simulink model "heli_q8"  (R2014a)
settings: Solver=ode1  StartTime=0.0  StopTime=inf  FixedStep=0.002  RelTol=1e-3
PostLoadFcn:
  | qc_set_target_type(getConfigSet(bdroot, 'QUARC Default Target Configuration'));
values from neighbouring files (symbols this model uses):
  A_p4p2 = [0 0 0 0 0 -0.926877316308 1 0 0 0 0 0 ... (36 elements, 6x6)]    [heli_v5.mat]    (also in init_heli.m = [)
  B_p4p2 = [0  0; 0  0.61746031746; 0  0; 0.0993637376927  0; 0  0; 0  0]    [heli_v5.mat]    (also in init_heli.m = [)
  C_p4p2 = [1 0 0 0 0 0 0 1 0 0 0 0 ... (18 elements, 3x6)]    [heli_v5.mat]    (also in init_heli.m = [)
  Joystick_gain_x = 1    [heli.mat]    (also in heli_v2.mat; heli_v3.mat; heli_v4.mat; heli_v5.mat)
  Joystick_gain_y = -1    [heli.mat]    (also in heli_v2.mat; heli_v3.mat; heli_v4.mat; heli_v5.mat)
  K_p3p2 = [0  0  10; 3.16227766017  3.35303639847  0]    [heli_v4.mat]    (also in heli_v5.mat = [0  0  31.6227766017; 3.16227766017  3.35303639847  0]; init_heli.m = lqr(A_p3p1,B_p3p1,Q_p3p2,R_p3p2))
  K_p3p3 = [3.11100011502e-16  -3.0775394805e-16  10.9602950373  -3.30376513683e-16  -1; 4.20040589293  3.82170483266  -1.91242655394e-15  -1  -1.23212746659e-16]    [heli_v4.mat]    (also in heli_v5.mat = [-5.30623224306e-17  4.08389146172e-16  32.3265792615  1.739; init_heli.m = lqr(A_p3p3,B_p3p3,Q_p3p3,R_p3p3))
  K_pd = 1    [heli_v2.mat]    (also in heli_v3.mat = 11.6606683805; heli_v4.mat = 11.6606683805; heli_v5.mat = 11.6606683805; matlab_v4.mat = 11.6606683805)
  K_pp = 1    [heli_v2.mat]    (also in heli_v3.mat = 20.9892030848; heli_v4.mat = 20.9892030848; heli_v5.mat = 20.9892030848; matlab_v4.mat = 20.9892030848)
  K_rp = 10    [heli_v3.mat]    (also in heli_v4.mat = 3; heli_v5.mat = 3; matlab_v4.mat = 3)
  L = [5.92554151514 9.30695114405 0.0303026409954 -0.158988846376 1.02705256088 2.3799077818 0.00310751540277 -0.175228041509 6.12526482605 9.80708337963 0.209399631745 0.659991765117 ... (18 elements, 6x3)]    [heli_v5.mat]    (also in init_heli.m = place(A_p4p2',C_p4p2',poles).')
  P_p3p2 = [0  10; 3.16227766017  0]    [heli_v4.mat]    (also in heli_v5.mat = [0  31.6227766017; 3.16227766017  0]; init_heli.m = inv(C_p3p1*inv(B_p3p1*K_p3p2-A_p3p1)*B_p3p1))
  P_p3p3 = [9.92153997111  9.06487564165e+16; 2.9174989874e+16  35.9409347137]    [heli_v4.mat]    (also in heli_v5.mat = [-5.30623224306e-17  32.3265792615; 3.49573681243  2.5377879; init_heli.m = inv(C_p3p1*inv(B_p3p1*K_p3p3(1:2,1:3) - A_p3p1)*B_p3p1))
  V_zero_offset = 6.4201    [heli_v4.mat]    (also in heli_v5.mat; init_heli.m)
undefined symbols (not defined in the file or in its folder): HIL, qc_get_step_size
libraries: simulink x9, simulink_extras x6, quarc_library x4
settings Model: SimulationMode=external  ExtModeTrigDuration=5000  Creator=Rchan  LastModifiedBy=magho
settings SolverCC: PositivePriorityOrder=on
settings DataIOCC: SignalLoggingSaveFormat=ModelDataLogs
settings OptimizationCC: ExpressionDepthLimit=2147483647  InitFltsAndDblsToZero=on
settings DebuggingCC: SaveWithParameterizedLinksMsg=none  UnderspecifiedInitializationDetection=Classic  MultiTaskDSMMsg=warning  MultiTaskCondExecSysMsg=none  MultiTaskRateTransMsg=warning  FcnCallInpInsideContextMsg=UseLocalSettings  StateNameClashWarn=warning
settings RTWCC: SystemTargetFile=quarc_win64.tlc  TemplateMakefile=quarc_default_tmf  Description=QUARC Win64 Target  ProcessScript=quarc_win64_make_rtw_hook
settings STFCustomTargetCC: CPPClassGenCompliant=on
settings GRTTargetCC: ParMdlRefBuildCompliant=off  CompOptLevelCompliant=off  CombineOutputUpdateFcns=off  MatFileLogging=off  GRTInterface=on  ExtMode=on  ExtModeMexFile=quarc_comm

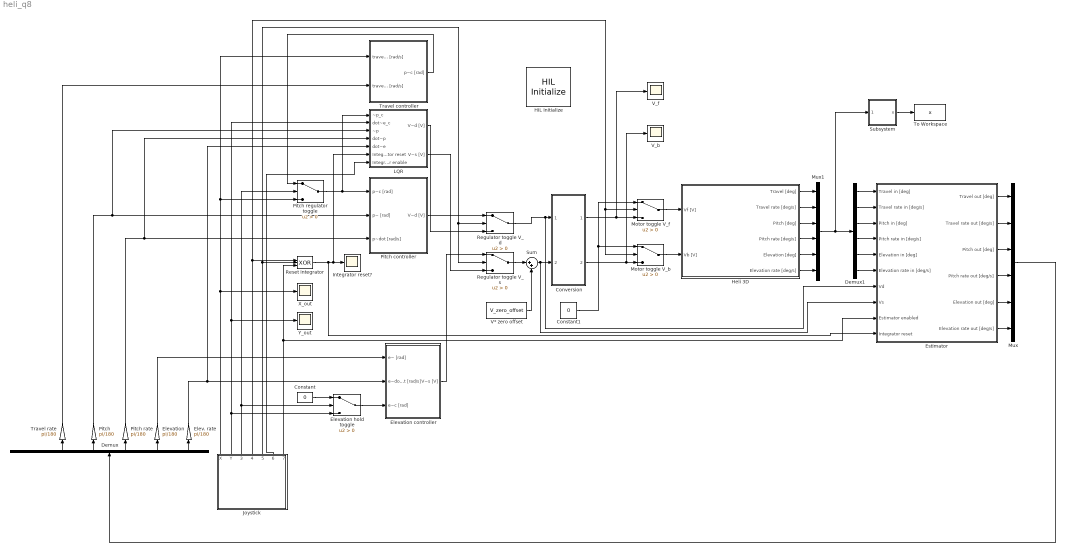
== system heli_q8 ==
  Constant : Constant  Value=0
  Constant1 : Constant  Value=0
  Conversion : Subsystem
  Demux : Demux  Outputs=6
  Demux1 : Demux  Outputs=6
  Elev. rate : Gain  Gain=pi/180
  Elevation : Gain  Gain=pi/180
  Elevation controller : Subsystem
  Elevation hold toggle : Switch  Criteria=u2 > Threshold
  Estimator : Subsystem
  HIL Initialize : quarc_library/Data Acquisition/Generic/Configuration/HIL Initialize  Priority=-99  object_name=HIL-1  board_type=q8_usb  board_number=0  board_options=update_rate=normal;decimation=1  exclusive=off  active=off  hardware_clocks=[0:2]  clock_modes=[]  initial_clock_frequencies=[]  set_clock_params_at_start=off  set_clock_params_at_switch_in=off  set_clock_frequencies_at_start=off  set_clock_frequencies_at_switch_in=off  analog_input_channels=[0:7]  analog_input_maximums=10  analog_input_minimums=-10  set_analog_input_params_at_start=on  set_analog_input_params_at_switch_in=off  analog_output_channels=[0:7]  analog_output_maximums=10  analog_output_minimums=-10  initial_analog_outputs=[0]  final_analog_outputs=[0]  watchdog_analog_outputs=0  set_analog_output_params_at_start=on  set_analog_output_params_at_switch_in=off  set_analog_outputs_at_start=on  set_analog_outputs_at_switch_in=off  set_analog_outputs_at_terminate=on  set_analog_outputs_at_switch_out=off  set_analog_outputs_on_watchdog=off  digital_input_channels=[]  digital_output_channels=[]  digital_output_configuration=[]  initial_digital_outputs=[1]  final_digital_outputs=[1]  watchdog_digital_outputs=[1]  set_digital_output_params_at_start=off  set_digital_output_params_at_switch_in=off  set_digital_outputs_at_start=on  set_digital_outputs_at_switch_in=off  set_digital_outputs_at_terminate=on  set_digital_outputs_at_switch_out=off  set_digital_outputs_on_watchdog=off  encoder_channels=[0:7]  quadrature=[4]  encoder_filter_frequency=[]  initial_encoder_counts=[0]  set_encoder_params_at_start=on  set_encoder_params_at_switch_in=off  set_encoder_counts_at_start=on  set_encoder_counts_at_switch_in=off  pwm_channels=[0:7]  pwm_modes=0  pwm_frequency=99.532799999999995e6/4095  pwm_configuration=[0]  pwm_alignment=[0]  pwm_polarity=[1]  pwm_leading_deadband=[0]  pwm_trailing_deadband=[0]  initial_pwm_outputs=[0]  final_pwm_outputs=[0]  watchdog_pwm_outputs=[0]  set_pwm_params_at_start=on  set_pwm_params_at_switch_in=off  set_pwm_outputs_at_start=on  set_pwm_outputs_at_switch_in=off  set_pwm_outputs_at_terminate=on  set_pwm_outputs_at_switch_out=off  set_pwm_outputs_on_watchdog=off  other_output_channels=[]  initial_other_outputs=[]  final_other_outputs=[]  watchdog_other_outputs=[]  set_other_outputs_at_start=off  set_other_outputs_at_switch_in=off  set_other_outputs_at_terminate=off  set_other_outputs_at_switch_out=off  set_other_outputs_on_watchdog=off
  Heli 3D : Subsystem
  Integrator reset? : Scope
      settings: TimeRange=10  YMin=-1  YMax=6.5  SaveName=ScopeData18
  Joystick : Subsystem
  LQR : Subsystem
  Motor toggle V_b : Switch  Criteria=u2 > Threshold
  Motor toggle V_f : Switch  Criteria=u2 > Threshold
  Mux : Mux  Inputs=6
  Mux1 : Mux  Inputs=6
  Pitch : Gain  Gain=pi/180
  Pitch controller : Subsystem
  Pitch rate : Gain  Gain=pi/180
  Pitch regulator toggle : Switch  Criteria=u2 > Threshold
  Regulator toggle V_d : Switch  Criteria=u2 > Threshold
  Regulator toggle V_s : Switch  Criteria=u2 > Threshold
  Reset integrator : Logic  Operator=XOR  Inputs=3  AllPortsSameDT=off  OutDataTypeStr=boolean
  Subsystem : Subsystem
  Sum : Sum  Inputs=|++
  To Workspace : ToWorkspace  VariableName=x  SaveFormat=Structure With Time  SampleTime=-1
  Travel controller : Subsystem
  Travel rate : Gain  Gain=pi/180
  "V* zero offset " : Constant  Value=V_zero_offset
  V_b : Scope
      settings: YMin=-7e+16  YMax=8e+16  SaveName=ScopeData17
  V_f : Scope
      settings: YMin=0  YMax=1.8e+15  SaveName=ScopeData16
  X_out : Scope
      settings: TimeRange=10  YMin=-1  YMax=6.5
  Y_out : Scope
      settings: YMax=8
  wires:
  Joystick/2(Y) -> Elevation hold toggle/3, Y_out/1, LQR/2(dot~e_c)
  Elev. rate/1 -> LQR/5(dot~e), Elevation controller/2(e~dot [rad/s])
  Elevation/1 -> Elevation controller/1(e~ [rad])
  Elevation controller/1(V~s [V]) -> Regulator toggle V_s/1
  Pitch/1 -> LQR/3(~p), Pitch controller/2(p~ [rad])
  Pitch rate/1 -> LQR/4(dot~p), Pitch controller/3(p~dot [rad/s])
  Constant/1 -> Elevation hold toggle/1
  Elevation hold toggle/1 -> Elevation controller/3(e~c [rad])
  Joystick/3(Travel Regulator Toggle) -> Elevation hold toggle/2, Pitch regulator toggle/2
  Pitch regulator toggle/1 -> Pitch controller/1(p~c [rad]), LQR/1(~p_c)
  Joystick/1(X) -> X_out/1, Pitch regulator toggle/3, Travel controller/1(travel rate_c [rad/s])
  Travel rate/1 -> Travel controller/2(travel rate [rad/s])
  Travel controller/1(p~c [rad]) -> Pitch regulator toggle/1
  Motor toggle V_b/1 -> Heli 3D/2(Vb [V])
  Motor toggle V_f/1 -> Heli 3D/1(Vf [V])
  Joystick/4(Motor Toggle) -> Motor toggle V_b/2, Motor toggle V_f/2, Reset integrator/1
  Conversion/2(Vb [V]) -> V_b/1, Motor toggle V_b/3
  Conversion/1(Vf [V]) -> V_f/1, Motor toggle V_f/3
  Constant1/1 -> Motor toggle V_f/1, Motor toggle V_b/1
  Regulator toggle V_d/1 -> Estimator/7(Vd), Conversion/1(Vd [V])
  Pitch controller/1(V~d [V]) -> Regulator toggle V_d/1
  Joystick/5(LQR toggle) -> Regulator toggle V_s/2, Regulator toggle V_d/2, Reset integrator/2
  LQR/2(V~s [V]) -> Regulator toggle V_s/3
  LQR/1(V~d [V]) -> Regulator toggle V_d/3
  Sum/1 -> Estimator/8(Vs), Conversion/2(Vs [V])
  Regulator toggle V_s/1 -> Sum/1
  "V* zero offset "/1 -> Sum/2
  Mux/1 -> Demux/1
  Demux/3 -> Pitch/1
  Demux/4 -> Pitch rate/1
  Demux/5 -> Elevation/1
  Demux/2 -> Travel rate/1
  Demux/6 -> Elev. rate/1
  Reset integrator/1 -> LQR/6(Integrator reset), Integrator reset?/1, Estimator/10(Integrator reset)
  Joystick/6(LQR integrator toggle) -> LQR/7(Integrator enable)
  Estimator/1(Travel out [deg]) -> Mux/1
  Estimator/3(Pitch out [deg]) -> Mux/3
  Estimator/4(Pitch rate out [deg/s]) -> Mux/4
  Estimator/5(Elevation out [deg]) -> Mux/5
  Estimator/6(Elevation rate out [deg/s]) -> Mux/6
  Estimator/2(Travel rate out [deg/s]) -> Mux/2
  Joystick/7(Estimator toggle) -> Reset integrator/3, Estimator/9("Estimator enabled ")
  Heli 3D/1(Travel [deg]) -> Mux1/1
  Heli 3D/2(Travel rate [deg/s]) -> Mux1/2
  Heli 3D/3(Pitch [deg]) -> Mux1/3
  Heli 3D/4(Pitch rate [deg/s]) -> Mux1/4
  Heli 3D/5(Elevation [deg]) -> Mux1/5
  Heli 3D/6(Elevation rate [deg/s]) -> Mux1/6
  Demux1/1 -> Estimator/1(Travel in [deg])
  Demux1/2 -> Estimator/2(Travel rate in [deg/s])
  Demux1/3 -> Estimator/3(Pitch in [deg])
  Demux1/4 -> Estimator/4(Pitch rate in [deg/s])
  Demux1/5 -> Estimator/5(Elevation in [deg])
  Demux1/6 -> Estimator/6(Elevation rate in [deg/s])
  Mux1/1 -> Subsystem/1(x_weird), Demux1/1
  Subsystem/1(x) -> To Workspace/1

== system heli_q8/Conversion ==
  Vd [V] : Inport
  Vs [V] : Inport  Port=2
  Add : Sum
  Back gain : Gain  Gain=0.5
  Front gain : Gain  Gain=0.5
  Subtract : Sum  Inputs=+-
  Vf [V] : Outport
  Vb [V] : Outport  Port=2
  wires:
  Vd [V]/1 -> Subtract/2, Add/1
  Vs [V]/1 -> Subtract/1, Add/2
  Subtract/1 -> Back gain/1
  Back gain/1 -> Vb [V]/1
  Add/1 -> Front gain/1
  Front gain/1 -> Vf [V]/1

== system heli_q8/Elevation controller ==
  e~ [rad] : Inport
  e~dot [rad/s] : Inport  Port=2
  e~c [rad] : Inport  Port=3
  Elevation controller : Subsystem
  Sum : Sum  Inputs=-+  SaturateOnIntegerOverflow=on  InputSameDT=on  OutDataTypeStr=Inherit: Same as first input
  V~s [V] : Outport  InitialOutput=0
  wires:
  Sum/1 -> Elevation controller/1(e~ [rad])
  Elevation controller/1(V~_s [V]) -> V~s [V]/1
  e~ [rad]/1 -> Sum/1
  e~dot [rad/s]/1 -> Elevation controller/2(e~_dot [rad/s])
  e~c [rad]/1 -> Sum/2

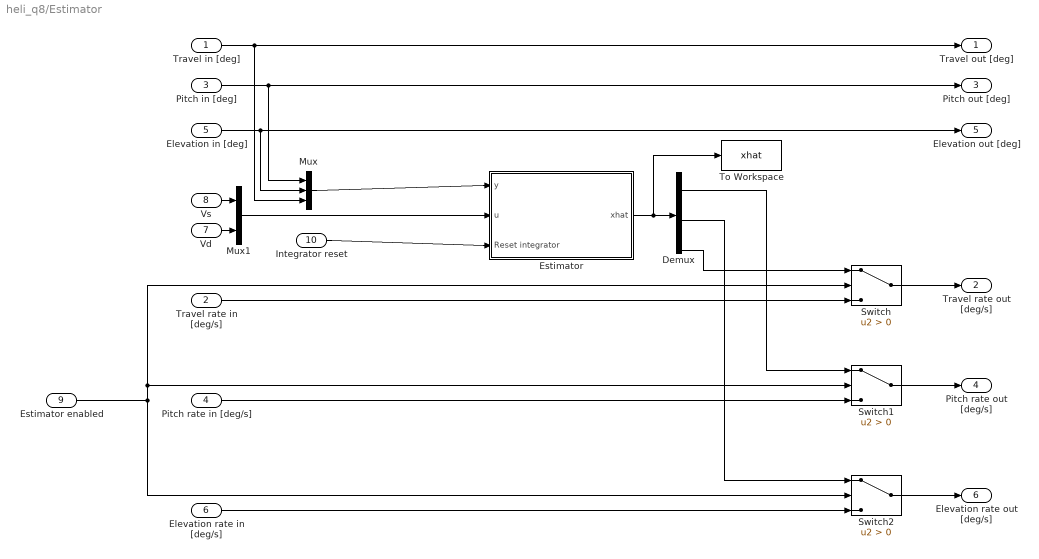
== system heli_q8/Estimator ==
  Travel in [deg] : Inport
  Travel rate in [deg/s] : Inport  Port=2
  Pitch in [deg] : Inport  Port=3
  Pitch rate in [deg/s] : Inport  Port=4
  Elevation in [deg] : Inport  Port=5
  Elevation rate in [deg/s] : Inport  Port=6
  Vd : Inport  Port=7
  Vs : Inport  Port=8
  "Estimator enabled " : Inport  Port=9
  Integrator reset : Inport  Port=10
  Demux : Demux  Outputs=6
  Estimator : Subsystem
  Mux : Mux  Inputs=3
  Mux1 : Mux  Inputs=2
  Switch : Switch  Criteria=u2 > Threshold
  Switch1 : Switch  Criteria=u2 > Threshold
  Switch2 : Switch  Criteria=u2 > Threshold
  To Workspace : ToWorkspace  VariableName=xhat  SaveFormat=Structure With Time  SampleTime=-1
  Travel out [deg] : Outport
  Travel rate out [deg/s] : Outport  Port=2
  Pitch out [deg] : Outport  Port=3
  Pitch rate out [deg/s] : Outport  Port=4
  Elevation out [deg] : Outport  Port=5
  Elevation rate out [deg/s] : Outport  Port=6
  wires:
  Travel in [deg]/1 -> Travel out [deg]/1, Mux/3
  Pitch in [deg]/1 -> Mux/1, Pitch out [deg]/1
  Elevation in [deg]/1 -> Elevation out [deg]/1, Mux/2
  Travel rate in [deg/s]/1 -> Switch/3
  Pitch rate in [deg/s]/1 -> Switch1/3
  Elevation rate in [deg/s]/1 -> Switch2/3
  Switch1/1 -> Pitch rate out [deg/s]/1
  Switch/1 -> Travel rate out [deg/s]/1
  Switch2/1 -> Elevation rate out [deg/s]/1
  "Estimator enabled "/1 -> Switch2/2, Switch/2, Switch1/2
  Mux/1 -> Estimator/1(y)
  Integrator reset/1 -> Estimator/3(Reset integrator)
  Vd/1 -> Mux1/2
  Vs/1 -> Mux1/1
  Mux1/1 -> Estimator/2(u)
  Estimator/1(xhat) -> To Workspace/1, Demux/1
  Demux/2 -> Switch1/1
  Demux/4 -> Switch2/1
  Demux/6 -> Switch/1

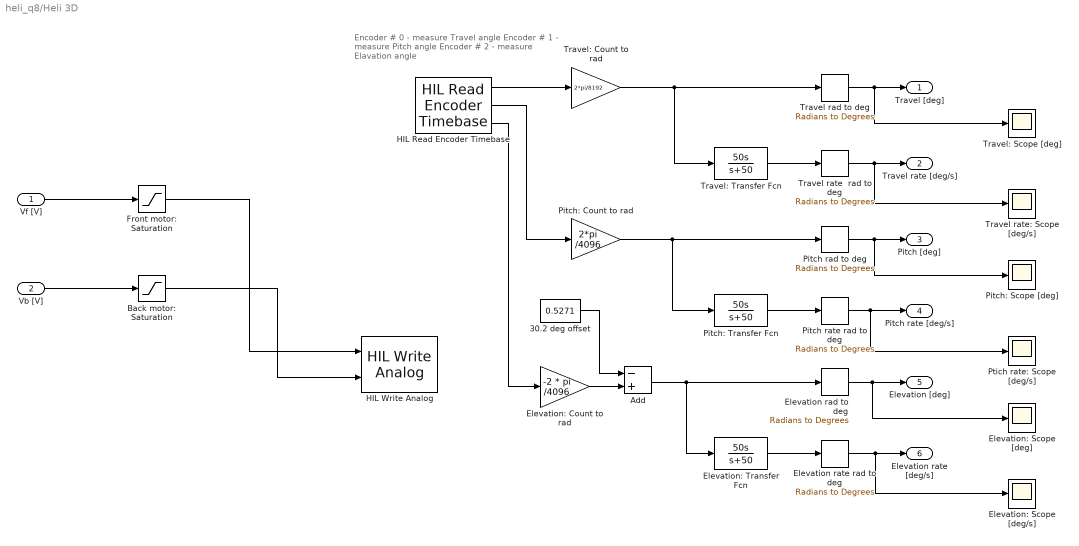
== system heli_q8/Heli 3D ==
  note: Encoder # 0 - measure Travel angle
      | Encoder # 1 - measure Pitch angle
      | Encoder # 2 - measure Elavation angle
  Vf [V] : Inport
  Vb [V] : Inport  Port=2
  30.2 deg offset : Constant  Value=0.5271
  Add : Sum  Inputs=-+
  Back motor: Saturation : Saturate  UpperLimit=5  LowerLimit=-5
  Elevation rad to deg : simulink_extras/Transformations/Radians to Degrees
  Elevation rate rad to deg : simulink_extras/Transformations/Radians to Degrees
  Elevation: Count to rad : Gain  Gain=-2 * pi /4096
  Elevation: Scope [deg/s] : Scope
      settings: YMin=-15  YMax=15  SaveName=ScopeData13
  Elevation: Scope [deg] : Scope
      settings: YMin=-32.5  YMax=0  SaveName=ScopeData12
  Elevation: Transfer Fcn : TransferFcn  Numerator=[50 0]  Denominator=[1 50]
  Front motor: Saturation : Saturate  UpperLimit=5  LowerLimit=-5
  HIL Read Encoder Timebase : quarc_library/Data Acquisition/Generic/Timebases/HIL Read Encoder Timebase  object_name=HIL-1  clock=0  channels=[0:2]  samples_in_buffer=max(ceil(1/qc_get_step_size), 1)  active=on  vector_output=off  data_type_mode=Inherit via back propagation  data_type=double
  HIL Write Analog : quarc_library/Data Acquisition/Generic/Immediate I//O/HIL Write Analog  object_name=HIL-1  channels=[0:1]  sample_time=-1  active=off  vector_input=off
  Pitch rad to deg : simulink_extras/Transformations/Radians to Degrees
  Pitch rate rad to deg : simulink_extras/Transformations/Radians to Degrees
  Pitch: Count to rad : Gain  Gain=2*pi /4096
  Pitch: Scope [deg] : Scope
      settings: YMin=-0.3  YMax=1  SaveName=ScopeData10
  Pitch: Transfer Fcn : TransferFcn  Numerator=[50 0]  Denominator=[1 50]
  Ptich rate: Scope [deg/s] : Scope
      settings: YMin=-15  YMax=15  SaveName=ScopeData11
  Travel rad to deg : simulink_extras/Transformations/Radians to Degrees
  Travel rate  rad to deg : simulink_extras/Transformations/Radians to Degrees
  Travel rate: Scope [deg/s] : Scope
      settings: YMin=-3.5  YMax=3  SaveName=ScopeData9
  Travel: Count to rad : Gain  Gain=2*pi/8192
  Travel: Scope [deg] : Scope
      settings: YMin=-2.75  YMax=0.5  SaveName=ScopeData8
  Travel: Transfer Fcn : TransferFcn  Numerator=[50 0]  Denominator=[1 50]
  Travel [deg] : Outport
  Travel rate [deg/s] : Outport  Port=2
  Pitch [deg] : Outport  Port=3
  Pitch rate [deg/s] : Outport  Port=4
  Elevation [deg] : Outport  Port=5
  Elevation rate [deg/s] : Outport  Port=6
  wires:
  HIL Read Encoder Timebase/1 -> Travel: Count to rad/1
  HIL Read Encoder Timebase/2 -> Pitch: Count to rad/1
  Travel: Count to rad/1 -> Travel: Transfer Fcn/1, Travel rad to deg/1
  Travel: Transfer Fcn/1 -> Travel rate  rad to deg/1
  Pitch: Count to rad/1 -> Pitch: Transfer Fcn/1, Pitch rad to deg/1
  Pitch: Transfer Fcn/1 -> Pitch rate rad to deg/1
  Elevation: Transfer Fcn/1 -> Elevation rate rad to deg/1
  Travel rad to deg/1 -> Travel: Scope [deg]/1, Travel [deg]/1
  Travel rate  rad to deg/1 -> Travel rate: Scope [deg/s]/1, Travel rate [deg/s]/1
  Pitch rad to deg/1 -> Pitch: Scope [deg]/1, Pitch [deg]/1
  Pitch rate rad to deg/1 -> Ptich rate: Scope [deg/s]/1, Pitch rate [deg/s]/1
  Elevation rad to deg/1 -> Elevation: Scope [deg]/1, Elevation [deg]/1
  Elevation rate rad to deg/1 -> Elevation: Scope [deg/s]/1, Elevation rate [deg/s]/1
  Vf [V]/1 -> Front motor: Saturation/1
  Vb [V]/1 -> Back motor: Saturation/1
  Front motor: Saturation/1 -> HIL Write Analog/1
  Back motor: Saturation/1 -> HIL Write Analog/2
  HIL Read Encoder Timebase/3 -> Elevation: Count to rad/1
  Elevation: Count to rad/1 -> Add/2
  Add/1 -> Elevation rad to deg/1, Elevation: Transfer Fcn/1
  30.2 deg offset/1 -> Add/1

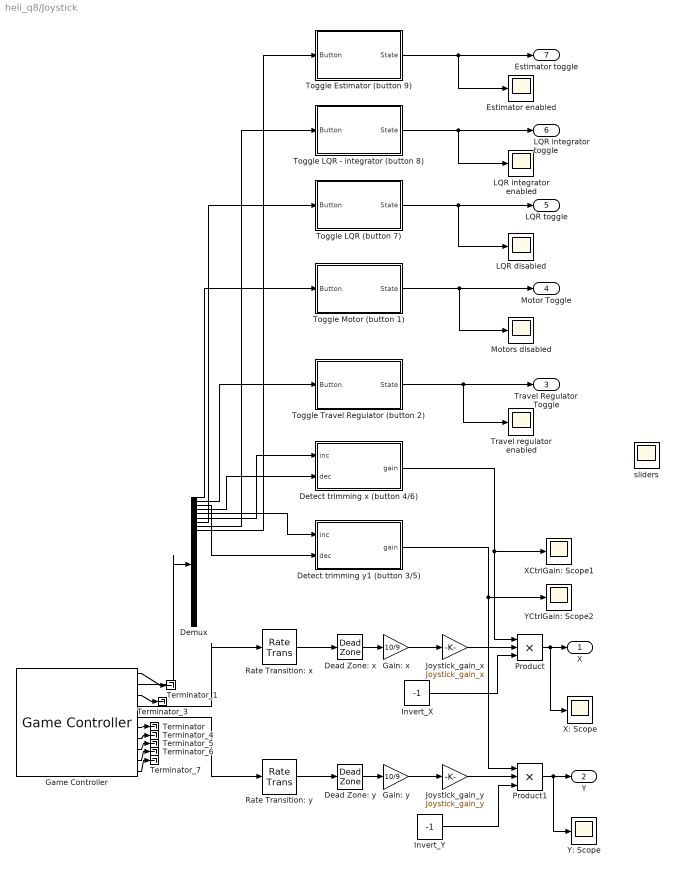
== system heli_q8/Joystick ==
  Dead Zone: x : DeadZone  LowerValue=-0.1  UpperValue=0.1  SaturateOnIntegerOverflow=on
  Dead Zone: y : DeadZone  LowerValue=-0.1  UpperValue=0.1  SaturateOnIntegerOverflow=on
  Demux : Demux  Outputs=32
  Detect trimming x (button 4/6) : Subsystem
  Detect trimming y1 (button 3/5) : Subsystem
  Estimator enabled : Scope
      settings: YMin=0.95  YMax=1.05  SaveName=ScopeData22
  Gain: x : Gain  Gain=10/9
  Gain: y : Gain  Gain=10/9
  Game Controller : quarc_library/Devices/Peripherals/Target/Game Controller  controller=1  buffer_size=12  deadzone=[]  saturation=[]  sample_time=max(qc_get_step_size, 0.01)  auto_center=off  enabled=on
  Invert_X : Constant  Value=-1
  Invert_Y : Constant  Value=-1
  Joystick_gain_x : Gain  Gain=Joystick_gain_x
  Joystick_gain_y : Gain  Gain=Joystick_gain_y
  LQR disabled : Scope
      settings: YMin=0.95  YMax=1.05  SaveName=ScopeData15
  LQR integrator enabled : Scope
      settings: YMin=0.95  YMax=1.05  SaveName=ScopeData21
  Motors disabled : Scope
      settings: YMin=0.95  YMax=1.05  SaveName=ScopeData6
  Product : Product  Inputs=3
  Product1 : Product  Inputs=3
  Rate Transition: x : RateTransition
  Rate Transition: y : RateTransition
  Terminator : Terminator
  Terminator_{1,3..7} (6 alike) : Terminator
  Toggle Estimator (button 9) : Subsystem
  Toggle LQR (button 7) : Subsystem
  Toggle LQR - integrator (button 8) : Subsystem
  Toggle Motor (button 1) : Subsystem
  Toggle Travel Regulator (button 2) : Subsystem
  Travel regulator enabled : Scope
      settings: YMin=0.95  YMax=1.05  SaveName=ScopeData14
  X: Scope : Scope
      settings: YMin=-1  YMax=1  SaveName=ScopeData7
  XCtrlGain: Scope1 : Scope
      settings: YMin=0  YMax=10  SaveName=ScopeData3
  Y: Scope : Scope
      settings: YMin=-10  YMax=10  SaveName=ScopeData5
  YCtrlGain: Scope2 : Scope
      settings: YMin=0  YMax=1.75  SaveName=ScopeData4
  sliders : Scope
      settings: YMin=-1  YMax=1  SaveName=ScopeData2
  X : Outport
  Y : Outport  Port=2
  Travel Regulator Toggle : Outport  Port=3
  Motor Toggle : Outport  Port=4
  LQR toggle : Outport  Port=5
  LQR integrator toggle : Outport  Port=6
  Estimator toggle : Outport  Port=7
  wires:
  Rate Transition: y/1 -> Dead Zone: y/1
  Rate Transition: x/1 -> Dead Zone: x/1
  Game Controller/5 -> Rate Transition: y/1
  Game Controller/4 -> Rate Transition: x/1
  Game Controller/1 -> Terminator_1/1
  Game Controller/7 -> Terminator_4/1
  Game Controller/8 -> Terminator_5/1
  Game Controller/9 -> Terminator_6/1
  Game Controller/10 -> Terminator_7/1
  Game Controller/6 -> Terminator/1
  Dead Zone: x/1 -> Gain: x/1
  Dead Zone: y/1 -> Gain: y/1
  Gain: x/1 -> Joystick_gain_x/1
  Gain: y/1 -> Joystick_gain_y/1
  Game Controller/2 -> Demux/1
  Game Controller/3 -> Terminator_3/1
  Joystick_gain_x/1 -> Product/2
  Detect trimming x (button 4/6)/1(gain) -> XCtrlGain: Scope1/1, Product/1
  Product/1 -> X: Scope/1, X/1
  Joystick_gain_y/1 -> Product1/2
  Product1/1 -> Y: Scope/1, Y/1
  Detect trimming y1 (button 3/5)/1(gain) -> Product1/1, YCtrlGain: Scope2/1
  Invert_X/1 -> Product/3
  Demux/6 -> Detect trimming x (button 4/6)/1(inc)
  Demux/4 -> Detect trimming x (button 4/6)/2(dec)
  Demux/5 -> Detect trimming y1 (button 3/5)/1(inc)
  Demux/3 -> Detect trimming y1 (button 3/5)/2(dec)
  Invert_Y/1 -> Product1/3
  Demux/1 -> Toggle Motor (button 1)/1(Button)
  Toggle Travel Regulator (button 2)/1(State) -> Travel regulator enabled/1, Travel Regulator Toggle/1
  Demux/2 -> Toggle Travel Regulator (button 2)/1(Button)
  Toggle Motor (button 1)/1(State) -> Motors disabled/1, Motor Toggle/1
  Demux/7 -> Toggle LQR (button 7)/1(Button)
  Toggle LQR (button 7)/1(State) -> LQR disabled/1, LQR toggle/1
  Demux/8 -> Toggle LQR - integrator (button 8)/1(Button)
  Toggle LQR - integrator (button 8)/1(State) -> LQR integrator enabled/1, LQR integrator toggle/1
  Demux/9 -> Toggle Estimator (button 9)/1(Button)
  Toggle Estimator (button 9)/1(State) -> Estimator enabled/1, Estimator toggle/1

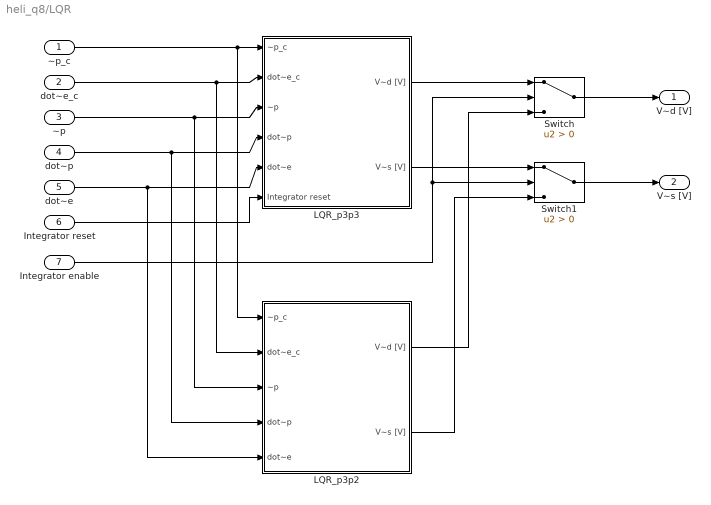
== system heli_q8/LQR ==
  ~p_c : Inport
  dot~e_c : Inport  Port=2
  ~p : Inport  Port=3
  dot~p : Inport  Port=4
  dot~e : Inport  Port=5
  Integrator reset : Inport  Port=6
  Integrator enable : Inport  Port=7
  LQR_p3p2 : Subsystem
  LQR_p3p3 : Subsystem
  Switch : Switch  Criteria=u2 > Threshold
  Switch1 : Switch  Criteria=u2 > Threshold
  V~d [V] : Outport
  V~s [V] : Outport  Port=2
  wires:
  ~p_c/1 -> LQR_p3p2/1(~p_c), LQR_p3p3/1(~p_c)
  dot~e_c/1 -> LQR_p3p2/2(dot~e_c), LQR_p3p3/2(dot~e_c)
  ~p/1 -> LQR_p3p2/3(~p), LQR_p3p3/3(~p)
  dot~p/1 -> LQR_p3p2/4(dot~p), LQR_p3p3/4(dot~p)
  dot~e/1 -> LQR_p3p2/5(dot~e), LQR_p3p3/5(dot~e)
  LQR_p3p3/1(V~d [V]) -> Switch/1
  Switch/1 -> V~d [V]/1
  Switch1/1 -> V~s [V]/1
  LQR_p3p3/2(V~s [V]) -> Switch1/1
  LQR_p3p2/1(V~d [V]) -> Switch/3
  LQR_p3p2/2(V~s [V]) -> Switch1/3
  Integrator reset/1 -> LQR_p3p3/6(Integrator reset)
  Integrator enable/1 -> Switch1/2, Switch/2

== system heli_q8/Pitch controller ==
  p~c [rad] : Inport
  p~ [rad] : Inport  Port=2
  p~dot [rad/s] : Inport  Port=3
  Add : Sum  Inputs=+-
  Add1 : Sum  Inputs=+-
  Gain : Gain  Gain=K_pp
  Gain1 : Gain  Gain=K_pd
  V~d [V] : Outport  InitialOutput=0
  wires:
  Add/1 -> V~d [V]/1
  p~dot [rad/s]/1 -> Gain1/1
  Gain1/1 -> Add/2
  p~c [rad]/1 -> Add1/1
  p~ [rad]/1 -> Add1/2
  Add1/1 -> Gain/1
  Gain/1 -> Add/1

== system heli_q8/Subsystem ==
  x_weird : Inport
  Demux2 : Demux  Outputs=6
  Mux2 : Mux  Inputs=6
  x : Outport
  wires:
  x_weird/1 -> Demux2/1
  Mux2/1 -> x/1
  Demux2/1 -> Mux2/5
  Demux2/2 -> Mux2/6
  Demux2/3 -> Mux2/1
  Demux2/4 -> Mux2/2
  Demux2/5 -> Mux2/3
  Demux2/6 -> Mux2/4

== system heli_q8/Travel controller ==
  travel rate_c [rad/s] : Inport
  travel rate [rad/s] : Inport  Port=2
  Add1 : Sum  Inputs=+-
  Gain : Gain  Gain=K_rp
  p~c [rad] : Outport  InitialOutput=0
  wires:
  Gain/1 -> p~c [rad]/1
  travel rate_c [rad/s]/1 -> Add1/2
  Add1/1 -> Gain/1
  travel rate [rad/s]/1 -> Add1/1

== system heli_q8/Elevation controller/Elevation controller ==
  e~ [rad] : Inport
  e~_dot [rad/s] : Inport  Port=2
  Integrator : Integrator  LimitOutput=on
  K_ed : Gain  Gain=12  SaturateOnIntegerOverflow=on  OutDataTypeStr=Inherit: Same as input  ParamDataTypeStr=Inherit: Same as input
  K_ei : Gain  Gain=5  SaturateOnIntegerOverflow=on  OutDataTypeStr=Inherit: Same as input  ParamDataTypeStr=Inherit: Same as input
  K_ep : Gain  Gain=15  SaturateOnIntegerOverflow=on  OutDataTypeStr=Inherit: Same as input  ParamDataTypeStr=Inherit: Same as input
  Sum : Sum  Inputs=++-  SaturateOnIntegerOverflow=on  InputSameDT=on  OutDataTypeStr=Inherit: Same as first input
  V~_s [V] : Outport  InitialOutput=0
  wires:
  K_ei/1 -> Integrator/1
  Integrator/1 -> Sum/1
  Sum/1 -> V~_s [V]/1
  e~_dot [rad/s]/1 -> K_ed/1
  K_ed/1 -> Sum/3
  K_ep/1 -> Sum/2
  e~ [rad]/1 -> K_ep/1, K_ei/1

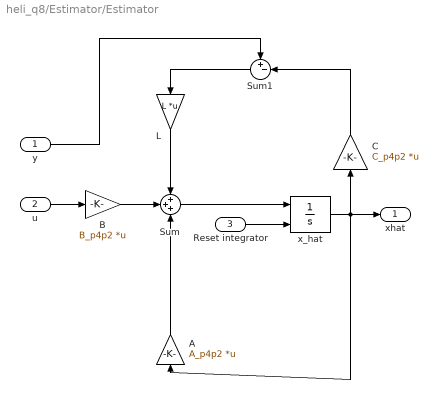
== system heli_q8/Estimator/Estimator ==
  y : Inport
  u : Inport  Port=2
  Reset integrator : Inport  Port=3
  A : Gain  Gain=A_p4p2  Multiplication=Matrix(K*u)
  B : Gain  Gain=B_p4p2  Multiplication=Matrix(K*u)
  C : Gain  Gain=C_p4p2  Multiplication=Matrix(K*u)
  L : Gain  Gain=L  Multiplication=Matrix(K*u)
  Sum : Sum  Inputs=+++
  Sum1 : Sum  Inputs=+-|
  x_hat : Integrator  ExternalReset=either
  xhat : Outport
  wires:
  x_hat/1 -> A/1, xhat/1, C/1
  Reset integrator/1 -> x_hat/2
  Sum/1 -> x_hat/1
  L/1 -> Sum/1
  y/1 -> Sum1/1
  C/1 -> Sum1/2
  Sum1/1 -> L/1
  A/1 -> Sum/3
  B/1 -> Sum/2
  u/1 -> B/1

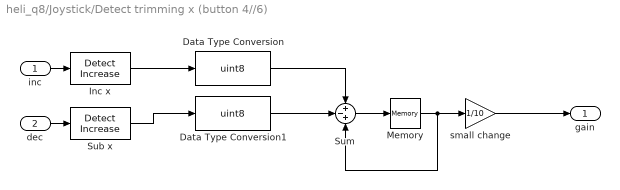
== system heli_q8/Joystick/Detect trimming x (button 4//6) ==
  inc : Inport
  dec : Inport  Port=2
  Data Type Conversion : DataTypeConversion  OutDataTypeStr=uint8
  Data Type Conversion1 : DataTypeConversion  OutDataTypeStr=uint8
  Inc x : simulink/Logic and Bit Operations/Detect Increase  vinit=0.0  InputProcessing=Inherited  OutDataTypeStr=boolean
  Memory : Memory  X0=20  InheritSampleTime=on
  Sub x : simulink/Logic and Bit Operations/Detect Increase  vinit=0.0  InputProcessing=Inherited  OutDataTypeStr=boolean
  Sum : Sum  Inputs=+-+
  small change : Gain  Gain=1/10
  gain : Outport
  wires:
  Sum/1 -> Memory/1
  Inc x/1 -> Data Type Conversion/1
  Memory/1 -> small change/1, Sum/3
  small change/1 -> gain/1
  Sub x/1 -> Data Type Conversion1/1
  inc/1 -> Inc x/1
  dec/1 -> Sub x/1
  Data Type Conversion/1 -> Sum/1
  Data Type Conversion1/1 -> Sum/2

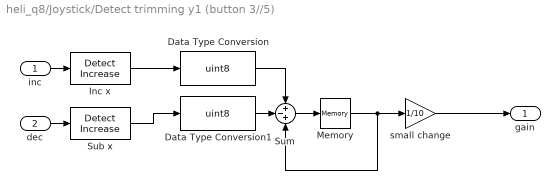
== system heli_q8/Joystick/Detect trimming y1 (button 3//5) ==
  inc : Inport
  dec : Inport  Port=2
  Data Type Conversion : DataTypeConversion  OutDataTypeStr=uint8
  Data Type Conversion1 : DataTypeConversion  OutDataTypeStr=uint8
  Inc x : simulink/Logic and Bit Operations/Detect Increase  vinit=0.0  InputProcessing=Inherited  OutDataTypeStr=boolean
  Memory : Memory  X0=15  InheritSampleTime=on
  Sub x : simulink/Logic and Bit Operations/Detect Increase  vinit=0.0  InputProcessing=Inherited  OutDataTypeStr=boolean
  Sum : Sum  Inputs=+-+
  small change : Gain  Gain=1/10
  gain : Outport
  wires:
  Sum/1 -> Memory/1
  Inc x/1 -> Data Type Conversion/1
  Memory/1 -> small change/1, Sum/3
  small change/1 -> gain/1
  Sub x/1 -> Data Type Conversion1/1
  inc/1 -> Inc x/1
  dec/1 -> Sub x/1
  Data Type Conversion/1 -> Sum/1
  Data Type Conversion1/1 -> Sum/2

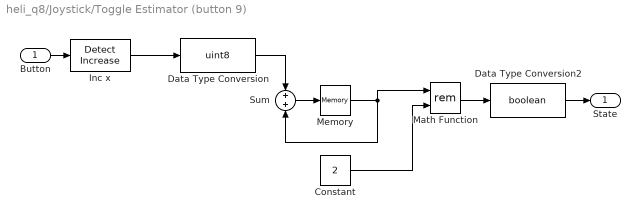
== system heli_q8/Joystick/Toggle Estimator (button 9) ==
  Button : Inport
  Constant : Constant  Value=2
  Data Type Conversion : DataTypeConversion  OutDataTypeStr=uint8
  Data Type Conversion2 : DataTypeConversion  OutDataTypeStr=boolean
  Inc x : simulink/Logic and Bit Operations/Detect Increase  vinit=0.0  InputProcessing=Inherited  OutDataTypeStr=boolean
  Math Function : Math  Operator=rem  SaturateOnIntegerOverflow=on
  Memory : Memory  X0=15  InheritSampleTime=on
  Sum : Sum
  State : Outport
  wires:
  Sum/1 -> Memory/1
  Inc x/1 -> Data Type Conversion/1
  Memory/1 -> Sum/2, Math Function/1
  Button/1 -> Inc x/1
  Data Type Conversion/1 -> Sum/1
  Constant/1 -> Math Function/2
  Math Function/1 -> Data Type Conversion2/1
  Data Type Conversion2/1 -> State/1

== system heli_q8/Joystick/Toggle LQR (button 7) ==
  Button : Inport
  Constant : Constant  Value=2
  Data Type Conversion : DataTypeConversion  OutDataTypeStr=uint8
  Data Type Conversion2 : DataTypeConversion  OutDataTypeStr=boolean
  Inc x : simulink/Logic and Bit Operations/Detect Increase  vinit=0.0  InputProcessing=Inherited  OutDataTypeStr=boolean
  Math Function : Math  Operator=rem  SaturateOnIntegerOverflow=on
  Memory : Memory  X0=15  InheritSampleTime=on
  Sum : Sum
  State : Outport
  wires:
  Sum/1 -> Memory/1
  Inc x/1 -> Data Type Conversion/1
  Memory/1 -> Sum/2, Math Function/1
  Button/1 -> Inc x/1
  Data Type Conversion/1 -> Sum/1
  Constant/1 -> Math Function/2
  Math Function/1 -> Data Type Conversion2/1
  Data Type Conversion2/1 -> State/1

== system heli_q8/Joystick/Toggle LQR - integrator (button 8) ==
  Button : Inport
  Constant : Constant  Value=2
  Data Type Conversion : DataTypeConversion  OutDataTypeStr=uint8
  Data Type Conversion2 : DataTypeConversion  OutDataTypeStr=boolean
  Inc x : simulink/Logic and Bit Operations/Detect Increase  vinit=0.0  InputProcessing=Inherited  OutDataTypeStr=boolean
  Math Function : Math  Operator=rem  SaturateOnIntegerOverflow=on
  Memory : Memory  X0=15  InheritSampleTime=on
  Sum : Sum
  State : Outport
  wires:
  Sum/1 -> Memory/1
  Inc x/1 -> Data Type Conversion/1
  Memory/1 -> Sum/2, Math Function/1
  Button/1 -> Inc x/1
  Data Type Conversion/1 -> Sum/1
  Constant/1 -> Math Function/2
  Math Function/1 -> Data Type Conversion2/1
  Data Type Conversion2/1 -> State/1

== system heli_q8/Joystick/Toggle Motor (button 1) ==
  Button : Inport
  Constant : Constant  Value=2
  Data Type Conversion : DataTypeConversion  OutDataTypeStr=uint8
  Data Type Conversion2 : DataTypeConversion  OutDataTypeStr=boolean
  Inc x : simulink/Logic and Bit Operations/Detect Increase  vinit=0.0  InputProcessing=Inherited  OutDataTypeStr=boolean
  Math Function : Math  Operator=rem  SaturateOnIntegerOverflow=on
  Memory : Memory  X0=15  InheritSampleTime=on
  Sum : Sum
  State : Outport
  wires:
  Sum/1 -> Memory/1
  Inc x/1 -> Data Type Conversion/1
  Memory/1 -> Sum/2, Math Function/1
  Button/1 -> Inc x/1
  Data Type Conversion/1 -> Sum/1
  Constant/1 -> Math Function/2
  Math Function/1 -> Data Type Conversion2/1
  Data Type Conversion2/1 -> State/1

== system heli_q8/Joystick/Toggle Travel Regulator (button 2) ==
  Button : Inport
  Constant : Constant  Value=2
  Data Type Conversion : DataTypeConversion  OutDataTypeStr=uint8
  Data Type Conversion2 : DataTypeConversion  OutDataTypeStr=boolean
  Inc x : simulink/Logic and Bit Operations/Detect Increase  vinit=0.0  InputProcessing=Inherited  OutDataTypeStr=boolean
  Math Function : Math  Operator=rem  SaturateOnIntegerOverflow=on
  Memory : Memory  X0=16  InheritSampleTime=on
  Sum : Sum
  State : Outport
  wires:
  Sum/1 -> Memory/1
  Inc x/1 -> Data Type Conversion/1
  Memory/1 -> Sum/2, Math Function/1
  Button/1 -> Inc x/1
  Data Type Conversion/1 -> Sum/1
  Constant/1 -> Math Function/2
  Math Function/1 -> Data Type Conversion2/1
  Data Type Conversion2/1 -> State/1

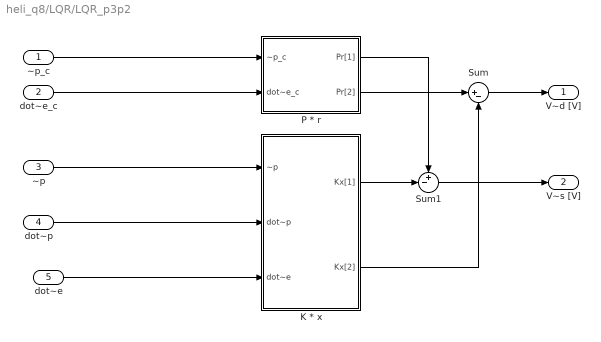
== system heli_q8/LQR/LQR_p3p2 ==
  ~p_c : Inport
  dot~e_c : Inport  Port=2
  ~p : Inport  Port=3
  dot~p : Inport  Port=4
  dot~e : Inport  Port=5
  K * x : Subsystem
  P * r : Subsystem
  Sum : Sum  Inputs=|+-
  Sum1 : Sum  Inputs=+-|
  V~d [V] : Outport
  V~s [V] : Outport  Port=2
  wires:
  dot~p/1 -> K * x/2(dot~p)
  ~p/1 -> K * x/1(~p)
  dot~e/1 -> K * x/3(dot~e)
  P * r/1(Pr[1]) -> Sum1/1
  P * r/2(Pr[2]) -> Sum/1
  K * x/2(Kx[2]) -> Sum/2
  ~p_c/1 -> P * r/1(~p_c)
  K * x/1(Kx[1]) -> Sum1/2
  dot~e_c/1 -> P * r/2(dot~e_c)
  Sum1/1 -> V~s [V]/1
  Sum/1 -> V~d [V]/1

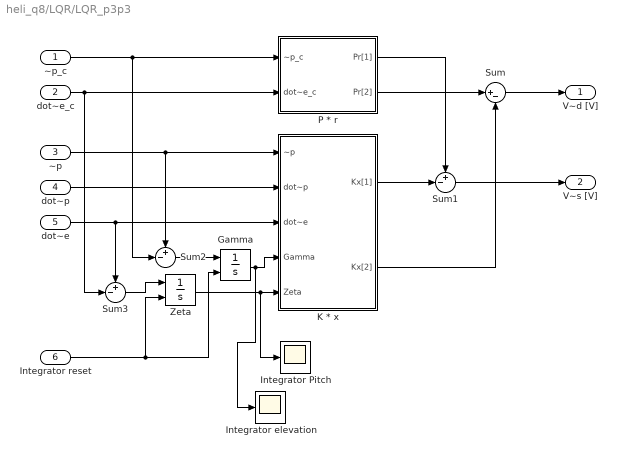
== system heli_q8/LQR/LQR_p3p3 ==
  ~p_c : Inport
  dot~e_c : Inport  Port=2
  ~p : Inport  Port=3
  dot~p : Inport  Port=4
  dot~e : Inport  Port=5
  Integrator reset : Inport  Port=6
  Gamma : Integrator  ExternalReset=either
  Integrator elevation : Scope
      settings: TimeRange=10  YMin=-1  YMax=6.5  SaveName=ScopeData20
  "Integrator Pitch " : Scope
      settings: TimeRange=10  YMin=-1  YMax=6.5  SaveName=ScopeData19
  K * x : Subsystem
  P * r : Subsystem
  Sum : Sum  Inputs=|+-
  Sum1 : Sum  Inputs=+-|
  Sum2 : Sum  Inputs=+-|
  Sum3 : Sum  Inputs=+-|
  Zeta : Integrator  ExternalReset=either
  V~d [V] : Outport
  V~s [V] : Outport  Port=2
  wires:
  dot~p/1 -> K * x/2(dot~p)
  ~p/1 -> Sum2/1, K * x/1(~p)
  dot~e/1 -> K * x/3(dot~e), Sum3/1
  P * r/1(Pr[1]) -> Sum1/1
  Gamma/1 -> Integrator elevation/1, K * x/4(Gamma)
  P * r/2(Pr[2]) -> Sum/1
  K * x/2(Kx[2]) -> Sum/2
  ~p_c/1 -> Sum2/2, P * r/1(~p_c)
  Zeta/1 -> "Integrator Pitch "/1, K * x/5(Zeta)
  K * x/1(Kx[1]) -> Sum1/2
  dot~e_c/1 -> Sum3/2, P * r/2(dot~e_c)
  Sum2/1 -> Gamma/1
  Sum1/1 -> V~s [V]/1
  Sum/1 -> V~d [V]/1
  Sum3/1 -> Zeta/1
  Integrator reset/1 -> Gamma/2, Zeta/2

== system heli_q8/LQR/LQR_p3p2/K * x ==
  ~p : Inport
  dot~p : Inport  Port=2
  dot~e : Inport  Port=3
  Demux : Demux  Outputs=2
  K * x : Gain  Gain=K_p3p2  Multiplication=Matrix(K*u) (u vector)
  Mux : Mux  Inputs=3
  Kx[1] : Outport
  Kx[2] : Outport  Port=2
  wires:
  Demux/1 -> Kx[1]/1
  Demux/2 -> Kx[2]/1
  K * x/1 -> Demux/1
  ~p/1 -> Mux/1
  dot~p/1 -> Mux/2
  dot~e/1 -> Mux/3
  Mux/1 -> K * x/1

== system heli_q8/LQR/LQR_p3p2/P * r ==
  ~p_c : Inport
  dot~e_c : Inport  Port=2
  Demux : Demux  Outputs=2
  Mux : Mux  Inputs=2
  P * r : Gain  Gain=P_p3p2  Multiplication=Matrix(K*u) (u vector)
  Pr[1] : Outport
  Pr[2] : Outport  Port=2
  wires:
  Demux/1 -> Pr[1]/1
  Demux/2 -> Pr[2]/1
  P * r/1 -> Demux/1
  Mux/1 -> P * r/1
  ~p_c/1 -> Mux/1
  dot~e_c/1 -> Mux/2

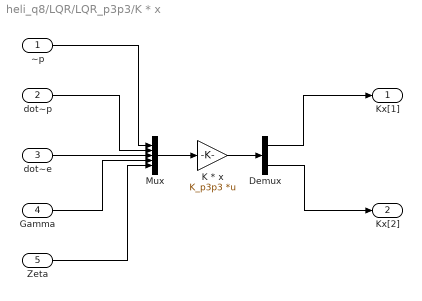
== system heli_q8/LQR/LQR_p3p3/K * x ==
  ~p : Inport
  dot~p : Inport  Port=2
  dot~e : Inport  Port=3
  Gamma : Inport  Port=4
  Zeta : Inport  Port=5
  Demux : Demux  Outputs=2
  K * x : Gain  Gain=K_p3p3  Multiplication=Matrix(K*u) (u vector)
  Mux : Mux  Inputs=5
  Kx[1] : Outport
  Kx[2] : Outport  Port=2
  wires:
  Demux/1 -> Kx[1]/1
  Demux/2 -> Kx[2]/1
  K * x/1 -> Demux/1
  ~p/1 -> Mux/1
  dot~p/1 -> Mux/2
  dot~e/1 -> Mux/3
  Mux/1 -> K * x/1
  Gamma/1 -> Mux/4
  Zeta/1 -> Mux/5

== system heli_q8/LQR/LQR_p3p3/P * r ==
  ~p_c : Inport
  dot~e_c : Inport  Port=2
  Demux : Demux  Outputs=2
  Mux : Mux  Inputs=2
  P * r : Gain  Gain=P_p3p3  Multiplication=Matrix(K*u) (u vector)
  Pr[1] : Outport
  Pr[2] : Outport  Port=2
  wires:
  Demux/1 -> Pr[1]/1
  Demux/2 -> Pr[2]/1
  P * r/1 -> Demux/1
  Mux/1 -> P * r/1
  ~p_c/1 -> Mux/1
  dot~e_c/1 -> Mux/2
